simulink model "Black_Box"  (R2016a)
settings: Solver=VariableStepAuto  StartTime=0.0  StopTime=10.0  RelTol=1e-3
values from neighbouring files (symbols this model uses):
  K = 651/12    (= 54.25)    [Model.m]    (also in PID_test.m = 96.2958333333; Rlocus.m = 0.0274)
  T = 0.014    [Model.m]    (also in PID_test.m = 0.12)
libraries: simulink x1
settings Model: Creator=Kristian  LastModifiedBy=Kristian

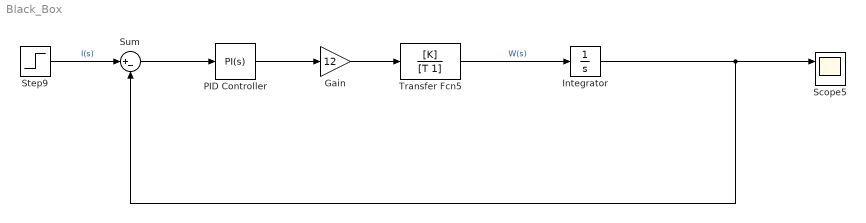
== system Black_Box ==
  Gain : Gain  Gain=12
  Integrator : Integrator
  PID Controller : simulink/Continuous/PID Controller  Controller=PI  TimeDomain=Continuous-time  SampleTime=-1  IntegratorMethod=Forward Euler  FilterMethod=Forward Euler  Form=Parallel  UseFilter=on  ControllerParametersSource=internal  P=1.44174860287022  I=11.4489443433005  D=0.0273396774002337  N=127212.148088975  InitialConditionSource=internal  InitialConditionForIntegrator=0  InitialConditionForFilter=0  ExternalReset=none  LimitOutput=off  UpperSaturationLimit=inf  LowerSaturationLimit=-inf  LinearizeAsGain=on  AntiWindupMode=none  Kb=1  TrackingMode=off  Kt=1  PParamMin=[]  PParamMax=[]  IParamMin=[]  IParamMax=[]  DParamMin=[]  DParamMax=[]  NParamMin=[]  NParamMax=[]  KbParamMin=[]  KbParamMax=[]  KtParamMin=[]  KtParamMax=[]  POutMin=[]  POutMax=[]  IOutMin=[]  IOutMax=[]  DOutMin=[]  DOutMax=[]  NOutMin=[]  NOutMax=[]  KbOutMin=[]  KbOutMax=[]  KtOutMin=[]  KtOutMax=[]  IntegratorOutMin=[]  IntegratorOutMax=[]  FilterOutMin=[]  FilterOutMax=[]  SumOutMin=[]  SumOutMax=[]  SumI1OutMin=[]  SumI1OutMax=[]  SumI2OutMin=[]  SumI2OutMax=[]  SumI3OutMin=[]  SumI3OutMax=[]  SumDOutMin=[]  SumDOutMax=[]  SaturationOutMin=[]  SaturationOutMax=[]  IntegratorContinuousStateAttributes=''  IntegratorStateMustResolveToSignalObject=off  IntegratorRTWStateStorageClass=Auto  FilterContinuousStateAttributes=''  FilterStateMustResolveToSignalObject=off  FilterRTWStateStorageClass=Auto  DifferentiatorICPrevScaledInput=0  DifferentiatorOutMin=[]  DifferentiatorOutMax=[]
  Scope5 : Scope  NumInputPorts=2
  Step9 : Step  SampleTime=0
  Sum : Sum  Inputs=|+-
  Transfer Fcn5 : TransferFcn  Numerator=[K]  Denominator=[T 1]
  wires:
  Gain/1 -> Transfer Fcn5/1
  Transfer Fcn5/1 -> Integrator/1  "W(s)"
  Integrator/1 -> Sum/2, Scope5/1
  PID Controller/1 -> Gain/1
  Sum/1 -> PID Controller/1
  Step9/1 -> Sum/1  "I(s)"
